simulink library "mech_stewart_control_equil_leg"  (Simulink 7.1)
undefined symbols (not defined in the file or in its folder): lower_leg_inertia, lower_leg_mass, upper_leg_inertia, upper_leg_mass
libraries: mblibv1 x7
settings Model: Creator=jwendlan  LastModifiedBy=batserve  ExtModeAutoUpdateStatusClock=off

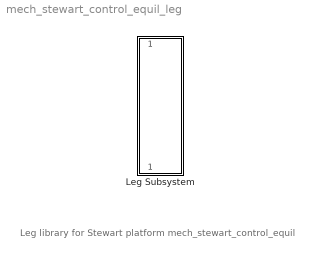
== system mech_stewart_control_equil_leg ==
  note: Leg library for Stewart platform
      | mech_stewart_control_equil
  Leg Subsystem : Subsystem  Orientation=down  mask{ln=1}
      mask prompts: ln "Leg Number"

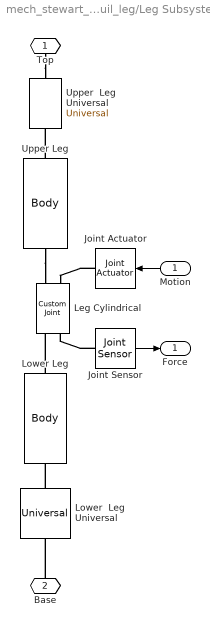
== system mech_stewart_control_equil_leg/Leg Subsystem ==
  Motion : Inport  Description=Applies a force (N) to the prismatic axis  Orientation=left  OutDataType=sfix(16)  OutScaling=2^0
  Joint Actuator : mblibv1/Sensors &  Actuators/Joint Actuator  Orientation=left  DialogController=MECH.DynMechDlgSource  SystemSampleTime=-1  PhysicalDomain=Mechanical  PortType=blob  ActuationStyle=Motion  AngleUnits=deg  ArcVelocityUnits=deg/s  ArcAccelerationUnits=deg/s^2  CoordPositionUnits=m  VelocityUnits=m/s  AccelerationUnits=m/s^2  ForceUnits=N  TorqueUnits=N-m  ActiveIO=off  Width=1  DialogClass=MechanicalActuatorBlock  Primitive=P1  ReferenceFrame=Absolute (INERTIAL)
  Joint Sensor : mblibv1/Sensors &  Actuators/Joint Sensor  DialogController=MECH.DynMechDlgSource  SystemSampleTime=-1  PhysicalDomain=Mechanical  PortType=blob  Muxed=on  Pose=off  Angle=on  AngleUnits=deg  ArcVelocity=off  ArcVelocityUnits=deg/s  ArcAcceleration=off  ArcAccelerationUnits=deg/s^2  CoordPosition=off  CoordPositionUnits=m  Velocity=off  VelocityUnits=m/s  Acceleration=off  AccelerationUnits=m/s^2  Quaternion=on  QuaternionDT=off  QuaternionDDT=off  QuaternionUnits=off  OutputVector=[ 1 ]  ActiveIO=off  Width=1  DialogClass=MechanicalSensorBlock  Primitive=P1  Force=on  ForceUnits=N  Torque=off  TorqueUnits=N-m  ReferenceFrame=Absolute (INERTIAL)  ReactionSensedSide=Base  ReactionReferenceFrame=Absolute (World)  ReactionForce=off  ReactionForceUnits=N  ReactionMoment=off  ReactionMomentUnits=N-m
  Leg Cylindrical : mblibv1/Joints/Custom Joint  Orientation=up  DialogController=MECH.DynMechDlgSource  PhysicalDomain=mechanical  SubClassName=custom_joint  LeftPortType=blob  RightPortType=blob  LConnTagsString=__newl0|SA1  RConnTagsString=__newr0|SA1  NumSAPorts=2  CutJoint=off  MarkAsCut=off  Primitives=revolute_prismatic  PrimitiveProps=R1$WORLD$cyl1(ln,:)$revolute#P1$WORLD$cyl1(ln,:)$prismatic  DialogClass=JointBlock  R1Axis=[0 0 1]  R2Axis=[]  R3Axis=[]  P1Axis=[]  P2Axis=[]  P3Axis=[]  SAxis=[]
  Lower Leg : mblibv1/Bodies/Body  Orientation=up  DialogController=MECH.DynMechDlgSource  PhysicalDomain=mechanical  SubClassName=Unknown  LeftPortType=workingframe  RightPortType=workingframe  LConnTagsString=CS1  RConnTagsString=CS3  DialogClass=MechanicalBodyBlock  Mass=lower_leg_mass  MassUnits=kg  InertiaUnits=kg*m^2  Inertia=lower_leg_inertia  Shape=Cylinder  ShapeDims=[1 1]  ShapeUnits=m  ShapeUse=false  Density=1  DensityUnits=kg/m^3  DensityUse=false  GraphicsMode=1  BodyColor=[0.5 0.5 0.5]  GraphicsObj=[]  AttachedToCS=1  CG=Left$CG$lower_leg(ln).origin$WORLD$WORLD$m$lower_leg(ln).rotation$3x3 Transform$deg$WORLD$false  WorkingFrames=Left$CS1$pos_base(ln,:)$WORLD$WORLD$m$lower_leg(ln).rotation$3x3 Transform$deg$WORLD$true#Right$CS3$(lower_leg(ln).end_point + upper_leg(ln).end_point)/2$WORLD$WORLD$m$lower_leg(ln).rotation$3x3 Transform$deg$WORLD$true#Right$CS2$lower_leg(ln).end_point$WORLD$WORLD$m$lower_leg(ln).rotation$3x3 Transform$deg$WORLD$false  CGPos=[0 0 0]  CGRot=[0 0 0]  CS0Pos=[]  CS0Rot=[]  CS1Pos=[0 0 0]  CS1Rot=[0 0 0]  CS2Pos=[0 0 0]  CS2Rot=[0 0 0]  CS3Pos=[]  CS3Rot=[]  CS4Pos=[]  CS4Rot=[]  CS5Pos=[]  CS5Rot=[]  CS6Pos=[]  CS6Rot=[]  CS7Pos=[]  CS7Rot=[]  CS8Pos=[]  CS8Rot=[]  CS9Pos=[]  CS9Rot=[]  CS10Pos=[]  CS10Rot=[]  CS11Pos=[]  CS11Rot=[]  CS12Pos=[]  CS12Rot=[]  CS13Pos=[]  CS13Rot=[]  CS14Pos=[]  CS14Rot=[]  CS15Pos=[]  CS15Rot=[]  CS16Pos=[]  CS16Rot=[]  CS17Pos=[]  CS17Rot=[]  CS18Pos=[]  CS18Rot=[]  CS19Pos=[]  CS19Rot=[]  CS20Pos=[]  CS20Rot=[]
  Lower  Leg Universal : mblibv1/Joints/Universal  Orientation=up  DialogController=MECH.DynMechDlgSource  PhysicalDomain=mechanical  SubClassName=Unknown  LeftPortType=blob  RightPortType=blob  LConnTagsString=__newl0  RConnTagsString=__newr0  NumSAPorts=0  CutJoint=off  MarkAsCut=off  Primitives=revolute_revolute  PrimitiveProps=R1$WORLD$rev1(ln,:)$revolute#R2$WORLD$rev2(ln,:)$revolute  DialogClass=JointBlock  R1Axis=[0 0 1]  R2Axis=[0 1 0]
  Upper Leg : mblibv1/Bodies/Body  Orientation=up  DialogController=MECH.DynMechDlgSource  PhysicalDomain=mechanical  SubClassName=Unknown  LeftPortType=workingframe  RightPortType=workingframe  LConnTagsString=CS3  RConnTagsString=CS2  DialogClass=MechanicalBodyBlock  Mass=upper_leg_mass  MassUnits=kg  InertiaUnits=kg*m^2  Inertia=upper_leg_inertia  Shape=Cylinder  ShapeDims=[1 1]  ShapeUnits=m  ShapeUse=false  Density=1  DensityUnits=kg/m^3  DensityUse=false  GraphicsMode=1  BodyColor=[0.5 0.5 0.5]  GraphicsObj=[]  AttachedToCS=1  CG=Left$CG$upper_leg(ln).origin$WORLD$WORLD$m$upper_leg(ln).rotation$3x3 Transform$deg$WORLD$false  WorkingFrames=Left$CS3$(lower_leg(ln).end_point + upper_leg(ln).end_point)/2$WORLD$WORLD$m$upper_leg(ln).rotation$3x3 Transform$deg$WORLD$true#Left$CS1$upper_leg(ln).end_point$WORLD$WORLD$m$upper_leg(ln).rotation$3x3 Transform$deg$WORLD$false#Right$CS2$pos_top(ln,:)$WORLD$WORLD$m$upper_leg(ln).rotation$3x3 Transform$deg$WORLD$true  CGPos=[0 0 0]  CGRot=[0 0 0]  CS0Pos=[]  CS0Rot=[]  CS1Pos=[0 0 0]  CS1Rot=[0 0 0]  CS2Pos=[0 0 0]  CS2Rot=[0 0 0]  CS3Pos=[]  CS3Rot=[]  CS4Pos=[]  CS4Rot=[]  CS5Pos=[]  CS5Rot=[]  CS6Pos=[]  CS6Rot=[]  CS7Pos=[]  CS7Rot=[]  CS8Pos=[]  CS8Rot=[]  CS9Pos=[]  CS9Rot=[]  CS10Pos=[]  CS10Rot=[]  CS11Pos=[]  CS11Rot=[]  CS12Pos=[]  CS12Rot=[]  CS13Pos=[]  CS13Rot=[]  CS14Pos=[]  CS14Rot=[]  CS15Pos=[]  CS15Rot=[]  CS16Pos=[]  CS16Rot=[]  CS17Pos=[]  CS17Rot=[]  CS18Pos=[]  CS18Rot=[]  CS19Pos=[]  CS19Rot=[]  CS20Pos=[]  CS20Rot=[]
  Upper  Leg Universal : mblibv1/Joints/Universal  Orientation=up  DialogController=MECH.DynMechDlgSource  PhysicalDomain=mechanical  SubClassName=Unknown  LeftPortType=blob  RightPortType=blob  LConnTagsString=__newl0  RConnTagsString=__newr0  NumSAPorts=0  CutJoint=off  MarkAsCut=off  Primitives=revolute_revolute  PrimitiveProps=R1$WORLD$rev3(ln,:)$revolute#R2$WORLD$rev4(ln,:)$revolute  DialogClass=JointBlock  R1Axis=[0 0 1]  R2Axis=[0 1 0]
  Top : PMIOPort  Orientation=down  Port=1  Side=Left
  Base : PMIOPort  Orientation=up  Port=2  Side=Right
  Force : Outport  Description=Senses position and velocity of the prismatic axis  OutDataType=sfix(16)  OutScaling=2^0
  wires:
  Motion/1 -> Joint Actuator/1
  Joint Sensor/1 -> Force/1
  connections:
  Lower  Leg Universal/RConn1 -- Lower Leg/LConn1
  Upper Leg/RConn1 -- Upper  Leg Universal/LConn1
  Top/RConn1 -- Upper  Leg Universal/RConn1
  Base/RConn1 -- Lower  Leg Universal/LConn1
  Joint Actuator/RConn1 -- Leg Cylindrical/RConn2
  Joint Sensor/LConn1 -- Leg Cylindrical/LConn2
  Lower Leg/RConn1 -- Leg Cylindrical/LConn1
  Upper Leg/LConn1 -- Leg Cylindrical/RConn1
